simulink model "sensorExpoler"  (R2026a)
settings: Solver=ode8  StopTime=inf  FixedStep=0.0005
undefined symbols (not defined in the file): Blocking, Discrete, Non, Time
libraries: fl_lib x11, nesl_utility x7, amg_usbconverter_n_connect_lib x2, ctrlSharedLib x1, dspstat3 x1, ee_lib x1
settings Model: Creator=pboon  LastModifiedBy=Passa

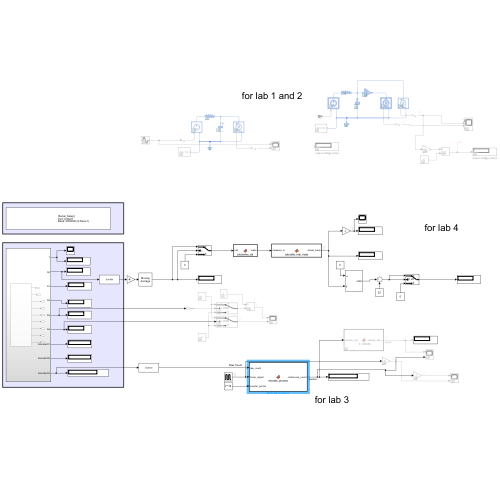
[thumbnail: Simulink's stored preview of the top-level diagram]
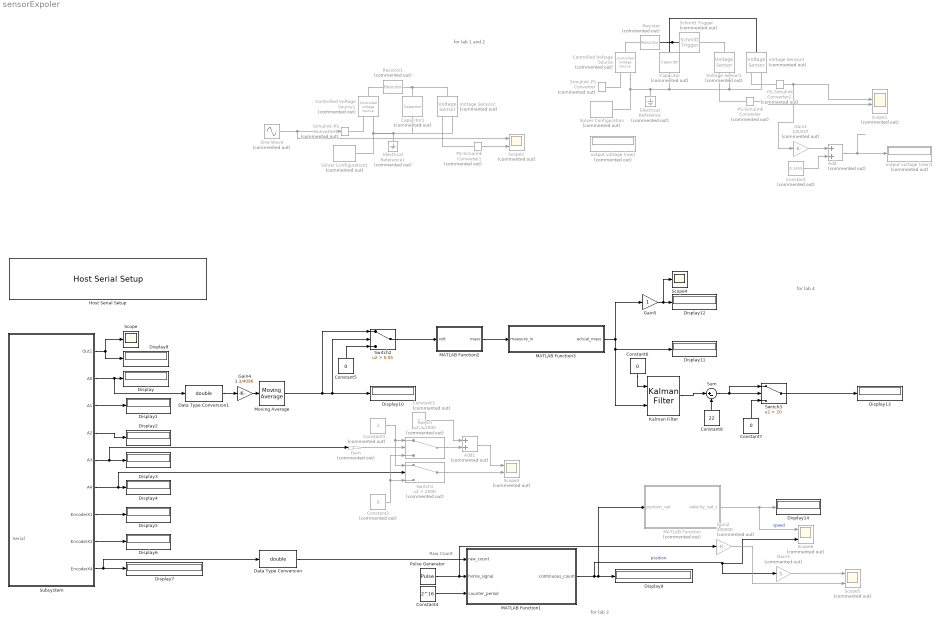
== system sensorExpoler ==
  note: for lab 1 and 2
  note: Raw Count
  note: Serial
  note: for lab 3
  note: for lab 4
  Add : Sum  Commented=on
  Add1 : Sum  Commented=on
  Capacitor : fl_lib/Electrical/Electrical Elements/Capacitor  Commented=on  c=15 uF  r=1e-6 Ohm  g=0 1/Ohm  i_specify=on  i_priority=None  i=0 A  i_nominal_specify=off  i_nominal_value=1  i_nominal_unit=A  v_specify=off  v_priority=None  v=0 V  v_nominal_specify=off  v_nominal_value=1  v_nominal_unit=V  vc_specify=off  vc_priority=High  vc=0 V  vc_nominal_specify=off  vc_nominal_value=1  vc_nominal_unit=V
  Capacitor1 : fl_lib/Electrical/Electrical Elements/Capacitor  Commented=on  c=470 uF  r=1e-6 Ohm  g=0 1/Ohm  i_specify=off  i_priority=None  i=0 A  i_nominal_specify=off  i_nominal_value=1  i_nominal_unit=A  v_specify=off  v_priority=None  v=0 V  v_nominal_specify=off  v_nominal_value=1  v_nominal_unit=V  vc_specify=off  vc_priority=High  vc=0 V  vc_nominal_specify=off  vc_nominal_value=1  vc_nominal_unit=V
  Constant : Constant  Commented=on  Value=0.2455
  Constant1 : Constant  Commented=on
  Constant2 : Constant  Commented=on  Value=0
  Constant3 : Constant  Commented=on  Value=2
  Constant4 : Constant  Value=2^16
  Constant5 : Constant  Value=0
  Constant6 : Constant  Value=0
  Constant7 : Constant  Value=0
  Constant8 : Constant  Value=22
  Controlled Voltage Source : fl_lib/Electrical/Electrical Sources/Controlled Voltage Source  Commented=on
  Controlled Voltage Source1 : fl_lib/Electrical/Electrical Sources/Controlled Voltage Source  Commented=on
  Data Type Conversion : DataTypeConversion  OutDataTypeStr=double  SaturateOnIntegerOverflow=off  RndMeth=Floor
  Data Type Conversion1 : DataTypeConversion  OutDataTypeStr=double  SaturateOnIntegerOverflow=off  RndMeth=Floor
  Display{,1..14} (15 alike) : Display
      Display10 settings: Decimation=5
      Display11 settings: Decimation=5
      Display12 settings: Decimation=5
      Display13 settings: Decimation=5
      Display14 settings: Decimation=5
  Electrical Reference : fl_lib/Electrical/Electrical Elements/Electrical Reference  Commented=on
  Electrical Reference1 : fl_lib/Electrical/Electrical Elements/Electrical Reference  Commented=on
  Gain : Gain  Commented=on  Gain=2
  Gain1 : Gain  Commented=on  Gain=1/0.037
  Gain2 : Gain  Commented=on  Gain=100000
  Gain3 : Gain  Commented=on  Gain=5
  Gain4 : Gain  Gain=3.3/4096
  Gain5 : Gain
  Host Serial Setup : amg_usbconverter_n_connect_lib/Host Serial Setup  conf=setup  port=<auto>  baudrate=2000000  databits=8  parity=None  stopbit=1  flowcontrol=None  transfer=Blocking  timeout=2  packetmode=Binary  initialvalues=[]  binheader='7E 7E'  binterminator='03 03'  porttype_double=0  porttype_single=1  porttype_int8=0  porttype_uint8=0  porttype_int16=0  porttype_uint16=0  porttype_int32=0  porttype_uint32=2  asciiformat='%d %u %x'  rx_asciiterminator="CRLF (0x0D 0x0A - \"\\r\\n\")"  tx_asciiterminator="CRLF (0x0D 0x0A - \"\\r\\n\")"  sampletime=-1  enablecustomportlabel=off  cinputportlabel=0  coutputportlabel=A  portpinstr=0  blockid=HostSerialSetup  inputporttype=[]  inputportwidth=[]  inputportlabel={}  outputporttype=[]  outputportwidth=[]  outputportlabel={}  compat=0  optionstring=[]  autoport='COM11'
  Kalman Filter : ctrlSharedLib/Kalman Filter  TimeDomain=Discrete-Time  UseCurrentEstimator=on  ModelSource=Individual A, B, C, D matrices  ModelSourceVariable=ss(0.95,1,1,0,1)  A=1  B=0  C=1  D=0  NumberOfStates=1  NumberOfInputs=1  NumberOfOutputs=1  Ts=-1  InitialEstimateSource=Dialog  X0=0  P0=10  UseK=off  UseGH=off  G=1  TimeInvariantG=on  H=0  TimeInvariantH=on  NumberOfProcessNoiseInputs=1  Q=0.1  TimeInvariantQ=on  R=10000  TimeInvariantR=on  N=0  TimeInvariantN=on  AddInputPort=on  AddEnablePort=off  OutputEstimatedY=off  OutputP=off
  MATLAB Function : MATLAB Function  Commented=on  TreatAsAtomicUnit=on
  MATLAB Function1 : MATLAB Function  TreatAsAtomicUnit=on
  MATLAB Function2 : MATLAB Function  TreatAsAtomicUnit=on
  MATLAB Function3 : MATLAB Function  TreatAsAtomicUnit=on
  Moving Average : dspstat3/Moving Average  Method=Sliding window  ForgettingFactorPort=off  SpecifyWindowLength=on  WindowLengthSource=Property  MaxWindowLength=20  WindowLength=50  OverlapLength=49  AllowArbitraryInputLength=off  ForgettingFactor=0.9  SimulateUsing=Interpreted execution
  PS-Simulink Converter : nesl_utility/PS-Simulink Converter  Commented=on  PhysicalDomain=network_engine_domain  SubClassName=ps_output  LeftPortType=input  RightPortType=output  PseudoPeriodic=off  Frequencies=[]  VectorFormat=inherit  Unit=inherit  AffineConversion=off
  PS-Simulink Converter1 : nesl_utility/PS-Simulink Converter  Commented=on  PhysicalDomain=network_engine_domain  SubClassName=ps_output  LeftPortType=input  RightPortType=output  PseudoPeriodic=off  Frequencies=[]  VectorFormat=inherit  Unit=inherit  AffineConversion=off
  PS-Simulink Converter2 : nesl_utility/PS-Simulink Converter  Commented=on  PhysicalDomain=network_engine_domain  SubClassName=ps_output  LeftPortType=input  RightPortType=output  PseudoPeriodic=off  Frequencies=[]  VectorFormat=inherit  Unit=inherit  AffineConversion=off
  Pulse Generator : DiscretePulseGenerator  PulseType=Time based  Period=6  PulseWidth=10
  Resistor : fl_lib/Electrical/Electrical Elements/Resistor  Commented=on  R=3317 Ohm  i_specify=off  i_priority=None  i=0 A  i_nominal_specify=off  i_nominal_value=1  i_nominal_unit=A  v_specify=off  v_priority=None  v=0 V  v_nominal_specify=off  v_nominal_value=1  v_nominal_unit=V
  Resistor1 : fl_lib/Electrical/Electrical Elements/Resistor  Commented=on  R=3317 Ohm  i_specify=off  i_priority=None  i=0 A  i_nominal_specify=off  i_nominal_value=1  i_nominal_unit=A  v_specify=off  v_priority=None  v=0 V  v_nominal_specify=off  v_nominal_value=1  v_nominal_unit=V
  Schmitt Trigger : ee_lib/Integrated Circuits/Logic/Schmitt Trigger  Commented=on  V_IL=1.5 V  V_IH=2.5 V  C_IN=5 pF  output_type=ee.enum.ic.outputType.linear  V_OL=0 V  V_OH=5 V  V_CC=5 V  V_meas=5 V  R_OUT=25 Ohm  R_OH=[25, 250] Ohm  I_OH=63 mA  R_OL=[30, 800] Ohm  I_OL=-45 mA  Delay=20 ns  Ron=5 Ohm  Vf=0.6 V  output_state=ee.enum.ic.initialState.low
  Scope : Scope
  Scope1 : Scope  Commented=on  NumInputPorts=4
      settings: ActiveDisplayYMinimum=-19.508526209310492  ActiveDisplayYMaximum=22.077675389777546
  Scope{2..3,5..6} (4 alike) : Scope  Commented=on  NumInputPorts=2
      Scope2 settings: ActiveDisplayYMinimum=-1.7674967613969836  ActiveDisplayYMaximum=1.7679475899562309  DataLoggingVariableName=ScopeData2
      Scope3 settings: ActiveDisplayYMinimum=-0.69984233895712267  ActiveDisplayYMaximum=3.4473209802051135  DataLoggingVariableName=ScopeData3
      Scope5 settings: ActiveDisplayYMinimum=-446039.56668591785  ActiveDisplayYMaximum=579588.43041542289  DataLoggingVariableName=ScopeData5
      Scope6 settings: ActiveDisplayYMinimum=-446039.56668591785  ActiveDisplayYMaximum=579588.43041542289  DataLoggingVariableName=ScopeData6
  Scope4 : Scope
      settings: ActiveDisplayYMinimum=-0.85467371033171546  ActiveDisplayYMaximum=7.6920633929854407  DataLoggingVariableName=ScopeData4
  Simulink-PS Converter : nesl_utility/Simulink-PS Converter  Commented=on  PhysicalDomain=network_engine_domain  SubClassName=ps_input  LeftPortType=input  RightPortType=output  PseudoPeriodic=off  Frequencies=[]  NoiseDistribution=none  NoiseParameters=[]  Unit=1  AffineConversion=off  FilteringAndDerivatives=filter  SimscapeFilterOrder=1  InputFilterTimeConstant=0.001  UdotUserProvided=0
  Simulink-PS Converter1 : nesl_utility/Simulink-PS Converter  Commented=on  PhysicalDomain=network_engine_domain  SubClassName=ps_input  LeftPortType=input  RightPortType=output  PseudoPeriodic=off  Frequencies=[]  NoiseDistribution=none  NoiseParameters=[]  Unit=1  AffineConversion=off  FilteringAndDerivatives=provide  SimscapeFilterOrder=1  InputFilterTimeConstant=0.001  UdotUserProvided=0
  Sine Wave : Sin  Commented=on  Frequency=0.5*2*pi  SampleTime=0
  Solver Configuration : nesl_utility/Solver Configuration  Commented=on  PhysicalDomain=network_engine_domain  SubClassName=solver  LeftPortType=input  RightPortType=generic  Tones=[]  Harmonics=[]  SimulateNoise=off  Profile=off  UseLocalSampling=off  EnableSwitchedLinearOptims=on  FrequencyDomain=off  UseCCode=off  RelTol=0.001  AbsTol=0.001  MinStep=1e-09  ToWorkspace=off  RevertToSquareIcSolve=off  NumHomotopyIterations=100  PhasorMode=off  PhasorModeNumHarmonics=1  ConsistencySolver=NEWTON_XTOL_AFTER_FTOL  CanonicalOrdering=CANONICAL  OptimizeIntermediates=OPTIMIZED  IndexReductionMethod=DerivativeReplacement  DoDC=off  ResidualTolerance=1e-09  ConsistencyTolSource=GLOBAL  ConsistencyAbsTol=0.001  ConsistencyRelTol=0.001  ConsistencyTolFactor=0.001  UseLocalSolver=on  LocalSolverChoice=NE_BACKWARD_EULER_ADVANCER  ResolveIndetEquations=on  FunctionEvalNumThread=1  LocalSolverSampleTime=0.001  DoFixedCost=off  MaxNonlinIter=3  MaxModeIter=2  ComputeImpulses=off  ImpulseIterations=2  LinearAlgebra=auto  LinearAlgebraNumThread=0  EquationFormulation=NE_TIME_EF  DelaysMemoryBudget=1024  AutomaticFiltering=on  FilteringTimeConstant=0.001  PartitionStorageMethod=AS_NEEDED  PartitionMemoryBudget=1024  PartitionMethod=ROBUST  MultibodyUseLocalSolver=off  MultibodyLocalSolverChoice=ODE1  MultibodyLocalSolverSampleTime=0.001
  Solver Configuration1 : nesl_utility/Solver Configuration  Commented=on  PhysicalDomain=network_engine_domain  SubClassName=solver  LeftPortType=input  RightPortType=generic  Tones=[]  Harmonics=[]  SimulateNoise=off  Profile=off  UseLocalSampling=off  EnableSwitchedLinearOptims=on  FrequencyDomain=off  UseCCode=off  RelTol=0.001  AbsTol=0.001  MinStep=1e-09  ToWorkspace=off  RevertToSquareIcSolve=off  NumHomotopyIterations=100  PhasorMode=off  PhasorModeNumHarmonics=1  ConsistencySolver=NEWTON_XTOL_AFTER_FTOL  CanonicalOrdering=CANONICAL  OptimizeIntermediates=OPTIMIZED  IndexReductionMethod=DerivativeReplacement  DoDC=off  ResidualTolerance=1e-09  ConsistencyTolSource=GLOBAL  ConsistencyAbsTol=0.001  ConsistencyRelTol=0.001  ConsistencyTolFactor=0.001  UseLocalSolver=off  LocalSolverChoice=NE_BACKWARD_EULER_ADVANCER  ResolveIndetEquations=on  FunctionEvalNumThread=1  LocalSolverSampleTime=0.001  DoFixedCost=off  MaxNonlinIter=3  MaxModeIter=2  ComputeImpulses=off  ImpulseIterations=2  LinearAlgebra=auto  LinearAlgebraNumThread=0  EquationFormulation=NE_TIME_EF  DelaysMemoryBudget=1024  AutomaticFiltering=on  FilteringTimeConstant=0.001  PartitionStorageMethod=AS_NEEDED  PartitionMemoryBudget=1024  PartitionMethod=ROBUST  MultibodyUseLocalSolver=off  MultibodyLocalSolverChoice=ODE1  MultibodyLocalSolverSampleTime=0.001
  Subsystem : Subsystem
  Sum : Sum  Inputs=|+-
  Switch : Switch  Commented=on  Criteria=u2 > Threshold  Threshold=2500  SaturateOnIntegerOverflow=off  InputSameDT=off
  Switch1 : Switch  Commented=on  Criteria=u2 > Threshold  Threshold=2500  SaturateOnIntegerOverflow=off  InputSameDT=off
  Switch2 : Switch  Criteria=u2 > Threshold  Threshold=0.05  SaturateOnIntegerOverflow=off  InputSameDT=off
  Switch3 : Switch  Criteria=u2 > Threshold  Threshold=20  SaturateOnIntegerOverflow=off  InputSameDT=off
  Voltage Sensor1 : fl_lib/Electrical/Electrical Sensors/Voltage Sensor  Commented=on
  Voltage Sensor2 : fl_lib/Electrical/Electrical Sensors/Voltage Sensor  Commented=on
  Voltage Sensor3 : fl_lib/Electrical/Electrical Sensors/Voltage Sensor  Commented=on
  output voltage (raw) : Display  Commented=on
  output voltage (raw)1 : Display  Commented=on
  wires:
  Subsystem/1(Out1) -> Display8/1, Scope/1
  Subsystem/2(A0) -> Data Type Conversion1/1, Display/1
  Subsystem/3(A1) -> Display1/1
  Subsystem/4(A2) -> Display2/1
  Subsystem/5(A3) -> Gain/1, Display3/1
  Subsystem/6(A4) -> Switch1/2, Display4/1
  Subsystem/7(EncoderX1) -> Display5/1
  Subsystem/8(EncoderX2) -> Display6/1
  Subsystem/9(EncoderX4) -> Data Type Conversion/1, Display7/1
  PS-Simulink Converter/1 -> Scope1/3
  PS-Simulink Converter1/1 -> Scope2/2
  Sine Wave/1 -> Scope2/1, Simulink-PS Converter1/1
  Gain1/1 -> Add/1
  Constant/1 -> Add/2
  Add/1 -> output voltage (raw)1/1
  PS-Simulink Converter2/1 -> Gain1/1, Scope1/2
  Switch/1 -> Add1/2
  Switch1/1 -> Scope3/2
  Constant1/1 -> Switch1/1, Switch/1
  Constant2/1 -> Switch/3, Switch1/3
  Constant3/1 -> Add1/1
  Add1/1 -> Scope3/1
  MATLAB Function1/1(continuous_count) -> Scope6/2, Gain3/1, MATLAB Function/1(position_rad), Display9/1  "position"
  Constant4/1 -> MATLAB Function1/3(counter_period)
  Pulse Generator/1 -> Gain2/1, MATLAB Function1/2(home_signal)
  Data Type Conversion/1 -> MATLAB Function1/1(raw_count)
  Gain/1 -> Switch/2
  Gain2/1 -> Scope5/2
  Gain3/1 -> Scope5/1
  Data Type Conversion1/1 -> Gain4/1
  Gain4/1 -> Moving Average/1
  MATLAB Function2/1(mass) -> MATLAB Function3/1(measure_in)
  Moving Average/1 -> Switch2/1, Switch2/2, Display10/1
  MATLAB Function3/1(actual_mass) -> Kalman Filter/2, Display11/1, Gain5/1
  Switch2/1 -> MATLAB Function2/1(volt)
  Constant5/1 -> Switch2/3
  Gain5/1 -> Scope4/1, Display12/1
  Constant6/1 -> Kalman Filter/1
  Constant7/1 -> Switch3/3
  Switch3/1 -> Display13/1
  Kalman Filter/1 -> Sum/1
  Sum/1 -> Switch3/1, Switch3/2
  Constant8/1 -> Sum/2
  MATLAB Function/1(velocity_rad_s) -> Scope6/1, Display14/1  "speed"
  connections:
  Simulink-PS Converter/RConn1 -- Controlled Voltage Source/RConn1
  Controlled Voltage Source/LConn1 -- Resistor/LConn1
  PS-Simulink Converter/LConn1 -- Voltage Sensor1/RConn1
  Voltage Sensor1/RConn2 -- Voltage Sensor3/RConn2 -- Capacitor/RConn1 -- Solver Configuration/RConn1 -- Controlled Voltage Source/RConn2 -- Electrical Reference/LConn1
  Controlled Voltage Source1/RConn2 -- Voltage Sensor2/RConn2 -- Capacitor1/RConn1 -- Electrical Reference1/LConn1 -- Solver Configuration1/RConn1
  Resistor1/RConn1 -- Voltage Sensor2/LConn1 -- Capacitor1/LConn1
  Controlled Voltage Source1/LConn1 -- Resistor1/LConn1
  PS-Simulink Converter1/LConn1 -- Voltage Sensor2/RConn1
  Simulink-PS Converter1/RConn1 -- Controlled Voltage Source1/RConn1
  Schmitt Trigger/LConn1 -- Resistor/RConn1 -- Voltage Sensor3/LConn1 -- Capacitor/LConn1
  Schmitt Trigger/RConn1 -- Voltage Sensor1/LConn1
  PS-Simulink Converter2/LConn1 -- Voltage Sensor3/RConn1

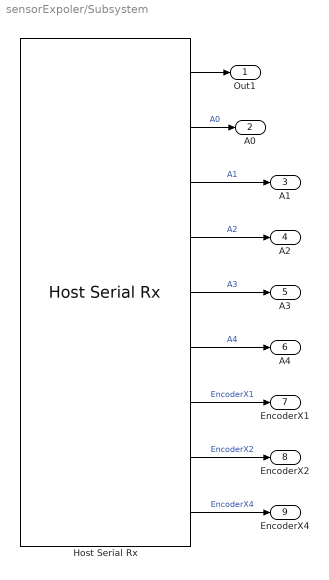
== system sensorExpoler/Subsystem ==
  Host Serial Rx : amg_usbconverter_n_connect_lib/Host Serial Rx  conf=rx  port=<auto>  baudrate=2000000  databits=8  parity=None  stopbit=1  flowcontrol=None  transfer=Non-Blocking  timeout=5  packetmode=Binary  enableinitialvalues=off  initialvalues=[]  binheader='25'  binterminator='4E 4E'  porttype_double=0  porttype_single=0  porttype_int8=0  porttype_uint8=0  porttype_int16=0  porttype_uint16=5  porttype_int32=0  porttype_uint32=3  asciiformat='%d,%f'  rx_asciiterminator="CRLF (0x0D 0x0A - \"\\r\\n\")"  tx_asciiterminator="CRLF (0x0D 0x0A - \"\\r\\n\")"  sampletime=0.0005  enablecustomportlabel=off  cinputportlabel=0  coutputportlabel=A  portpinstr=0  blockid=SubsystemHostSerialRx  inputporttype=[]  inputportwidth=[]  inputportlabel={}  outputporttype=[3 5 5 5 5 5 7 7 7]  outputportwidth=[1 1 1 1 1 1 1 1 1]  outputportlabel={'READY','uint16','uint16','uint16','uint16','uint16','uint32','uint32','uint32'}  compat=0  optionstring=[]  autoport='COM11'
  Out1 : Outport
  A0 : Outport  Port=2
  A1 : Outport  Port=3
  A2 : Outport  Port=4
  A3 : Outport  Port=5
  A4 : Outport  Port=6
  EncoderX1 : Outport  Port=7
  EncoderX2 : Outport  Port=8
  EncoderX4 : Outport  Port=9
  wires:
  Host Serial Rx/6 -> A4/1  "A4"
  Host Serial Rx/9 -> EncoderX4/1  "EncoderX4"
  Host Serial Rx/8 -> EncoderX2/1  "EncoderX2"
  Host Serial Rx/4 -> A2/1  "A2"
  Host Serial Rx/7 -> EncoderX1/1  "EncoderX1"
  Host Serial Rx/1 -> Out1/1
  Host Serial Rx/5 -> A3/1  "A3"
  Host Serial Rx/3 -> A1/1  "A1"
  Host Serial Rx/2 -> A0/1  "A0"

== matlab function sensorExpoler/MATLAB Function ==
  data: position_rad input; velocity_rad_s output
function velocity_rad_s = calc_velocity(position_rad)
    % กำหนด dt คงที่ตามรอบการรันของ Simulink (0.001 วินาที = 1 ms)
    dt = 0.0001; 
    
    % ค่าความหนืดของ Filter (ตั้งได้ตั้งแต่ 0 ถึง 0.99)
    % - ค่าใกล้ 0 = กราฟแกว่งเหมือนเดิม แต่ตอบสนองไว
    % - ค่าใกล้ 0.99 = กราฟเนียนกริบ แต่ความเร็วจะอัปเดตตามหลังของจริงนิดหน่อย (Delay)
    % ลองปรับเล่นดู แนะนำเริ่มที่ 0.85
    alpha = 0.85; 
    
    pos = double(position_rad);
    
    persistent prev_pos;
    persistent prev_vel_filtered;
    
    if isempty(prev_pos)
        prev_pos = pos;
        prev_vel_filtered = 0;
        velocity_rad_s = 0;
        return;
    end
    
    % 1. หาความเร็วดิบ (Raw Velocity) ที่จะแกว่งเป็นหนามๆ
    raw_vel = (pos - prev_pos) / dt;
    
    % 2. เอาความเร็วดิบมาเกลี่ยผ่าน Filter ให้กราฟเนียนขึ้น
    velocity_rad_s = (alpha * prev_vel_filtered) + ((1 - alpha) * raw_vel);
    
    % 3. จำค่าปัจจุบันไว้ใช้ในรอบ 0.001 วิ ถัดไป
    prev_pos = pos;
    prev_vel_filtered = velocity_rad_s;
end

== matlab function sensorExpoler/MATLAB Function2 ==
  data: volt input; mass output
function mass = piecewise_cal(volt)
    % 1. ค่าแรงดัน (Voltage) เฉลี่ยจากทั้ง 2 ชุด
    V = [0.03789, 0.18535, 0.54870, 0.85585, 1.18050, 1.51850, 1.83950, 2.17300, 2.50050, 2.82700];

    % 2. ค่าน้ำหนัก (Mass) เฉลี่ยจากทั้ง 2 ชุด
    M = [0.0, 307.0, 1302.5, 2288.5, 3272.0, 4246.0, 5209.5, 6203.0, 7188.0, 8149.5];

    mass = 0; % กำหนดค่าเริ่มต้น

    % 3. ตรวจสอบเงื่อนไขและหาช่วงที่แรงดันตกอยู่
    if volt <= V(1)
        mass = 0; % ถ้าต่ำกว่าศูนย์ให้โชว์ 0
    elseif volt >= V(end)
        % ถ้าน้ำหนักเกิน 8149.5 กรัม ให้ Extrapolate ต่อด้วยความชันของช่วงสุดท้าย
        m = (M(end) - M(end-1)) / (V(end) - V(end-1));
        c = M(end-1) - (m * V(end-1));
        mass = (m * volt) + c;
    else
        % ค้นหาช่วง Piecewise และคำนวณแบบ Linear Interpolation
        for i = 1:(length(V)-1)
            if volt >= V(i) && volt < V(i+1)
                m = (M(i+1) - M(i)) / (V(i+1) - V(i)); 
                c = M(i) - (m * V(i));                 
                mass = (m * volt) + c;                 
                break;
            end
        end
    end

    % 4. ดักจับค่าหน้าจอติดลบ
    if mass < 0
        mass = 0;
    end
end

== matlab function sensorExpoler/MATLAB Function3 ==
  data: measure_in input; actual_mass output
function actual_mass = calculate_real_mass(measure_in)
    % แกน X: ค่าน้ำหนักที่โปรแกรมอ่านได้ (Measure) 
    X = [10.585, 385.1, 403.4, 1147.0, 2159.0, 3165.0, 4127.0, 5118.5, 6107.5, 7122.5];
    
    % แกน Y: ค่าน้ำหนักตุ้มมาตรฐานของจริง (Actual Mass)
    Y = [0, 483, 500, 1460.5, 2427, 3408, 4398.5, 5384.5, 6378.5, 7386];

    actual_mass = 0; % ตั้งค่าเริ่มต้น

    % 1. ถ้าค่าน้อยกว่าจุดเริ่มต้น ให้เป็น 0
    if measure_in <= X(1)
        actual_mass = 0;
        
    % 2. ถ้าค่าเกินจุดสุดท้าย ให้ทะลุกราฟด้วยความชันของช่วงสุดท้าย
    elseif measure_in >= X(end)
        m = (Y(end) - Y(end-1)) / (X(end) - X(end-1));
        c = Y(end) - (m * X(end));
        actual_mass = (m * measure_in) + c;
        
    % 3. การหาความชัน (m) และคำนวณมวลกรัมของแต่ละช่วง (Piecewise)
    else
        for i = 1:(length(X)-1)
            % หาว่าค่าน้ำหนักที่อ่านได้ ตกอยู่ในช่วงไหน
            if measure_in >= X(i) && measure_in < X(i+1)
                
                % คำนวณความชัน (Gain = m) ของช่วงนั้น: m = dY / dX
                m = (Y(i+1) - Y(i)) / (X(i+1) - X(i));
                
                % คำนวณค่าชดเชย Offset (c) ของช่วงนั้น: c = Y - mX
                c = Y(i) - (m * X(i));
                
                % แปลงค่าออกเป็นมวลกรัมด้วยสมการเชิงเส้น: Y = mX + c
                actual_mass = (m * measure_in) + c;
                
                break; % คำนวณเสร็จให้หยุดลูป
            end
        end
    end

    % 4. ระบบป้องกันหน้าจอติดลบตอนไม่มีน้ำหนัก
    if actual_mass < 0
        actual_mass = 0;
    end
end

== matlab function sensorExpoler/MATLAB Function1 ==
  data: raw_count input; continuous_count output; home_signal input; counter_period input
function continuous_count = encoder_process(raw_count, home_signal, counter_period)
    curr_raw = double(raw_count);
    
    persistent prev_raw;
    persistent total_count;
    
    if isempty(prev_raw)
        prev_raw = curr_raw;
        total_count = 0;
    end
    
    diff = curr_raw - prev_raw;
    
    half_period = counter_period / 2;

    if diff < -half_period

        diff = diff + (counter_period + 1);
        
    elseif diff > half_period
        % เกิด Overflow ขาลง
        diff = diff - (counter_period + 1);
    end
    
    total_count = total_count + diff;
    
    % ----------------------------------------------------
    % 2. Homing Sequence Logic
    % ----------------------------------------------------

    if home_signal == 1
        total_count = 0;
    end
    
    % อัปเดตค่าดิบเพื่อใช้เปรียบเทียบในรอบถัดไป
    prev_raw = curr_raw;
    
    % ส่งออกค่า Count แบบต่อเนื่อง (สามารถนำไปแปลงเป็น Pulses, Radians, Velocity ต่อได้)
    continuous_count = total_count;
end
